simulink model "UpDownCounterOneState"  (R2025a)
settings: Solver=FixedStepDiscrete  StartTime=0.0  StopTime=Inf  RelTol=1e-3
libraries: simulink_extras x1
settings Model: PacingRate=1.500000  Creator=Soochan Kim  LastModifiedBy=Soochan Kim
settings OptimizationCC: BlockReduction=off  ConditionallyExecuteInputs=off  DefaultParameterBehavior=Inlined
settings DebuggingCC: AlgebraicLoopMsg=error
settings HardwareCC: ProdBitPerPointer=32.0  ProdBitPerSizeT=32.0  ProdBitPerPtrDiffT=32.0  ProdLargestAtomicFloat=None  ProdIntDivRoundTo=Undefined  ProdEndianess=Unspecified  ProdWordSize=32.0  ProdHWDeviceType=ASIC/FPGA->ASIC/FPGA  TargetBitPerPointer=64.0  TargetBitPerSizeT=64.0  TargetBitPerPtrDiffT=64.0  TargetLongLongMode=on  TargetIntDivRoundTo=Zero  TargetEndianess=LittleEndian  TargetWordSize=64.0  TargetHWDeviceType=Custom Processor->MATLAB Host Computer  ProdEqTarget=off

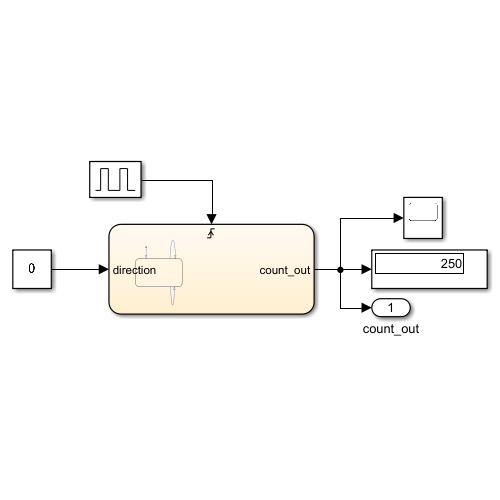
[thumbnail: Simulink's stored preview of the top-level diagram]
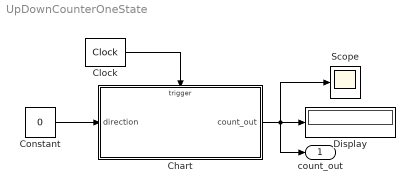
== system UpDownCounterOneState ==
  Chart : Stateflow chart  TreatAsAtomicUnit=on
  Clock : simulink_extras/Flip Flops/Clock  period=1
  Constant : Constant  Value=0
  Display : Display
  Scope : Scope
      settings: ActiveDisplayYMinimum=-31.124999999999993  ActiveDisplayYMaximum=280.125
  count_out : Outport  OutDataTypeStr=uint8  VectorParamsAs1DForOutWhenUnconnected=off
  wires:
  Chart/1(count_out) -> count_out/1, Scope/1, Display/1
  Clock/1 -> Chart/Trigger
  Constant/1 -> Chart/1(direction)

== stateflow chart UpDownCounterOneState/Chart ==
  settings: executeAtInitialization=1
  state CNT
  CNT -> CNT [order 1] : clk [direction == 1] {count = count + 1; count_out = count;}
  (default) -> CNT
  CNT -> CNT [order 2] : clk [direction == 0] {count = count - 1; count_out = count;}
  data: direction input; count_out output uint8; count local uint8 =0
  events: clk input RISING_EDGE_EVENT
